simulink model "iPMSM_EKF"  (R2023a)
settings: Solver=FixedStepAuto  StartTime=0.0  StopTime=10  FixedStep=0.0001  RelTol=1e-3  EnableMultiTasking=on
model workspace (MATLAB code in the model file + MAT data in the model file):
  cmdLim = Simulink.Parameter
  cmdLim.Value = 15
  cmdLim.Description = 'Limit for controlling the maximum surface command angle.'
  cmdLim.Min = 0
  cmdLim.Max = 90
  cmdLim.DocUnits = 'deg'
  dispGain = Simulink.Parameter
  dispGain.Value = 0.75
  dispGain.Description = 'Gain applied to the displacement error.'
  dispGain.Min = 0
  dispGain.Max = []
  dispGain.DocUnits = 'deg/sec/deg'
  dispLim = Simulink.Parameter
  dispLim.Value = 30
  dispLim.Description = 'Limit for controlling the maximum commanded angle.'
  dispLim.Min = 0
  dispLim.Max = 180
  dispLim.DocUnits = 'deg'
  intGain = Simulink.Parameter
  intGain.Value = 0.5
  intGain.Description = 'Gain applied to the integral error.'
  intGain.Min = 0
  intGain.Max = []
  intGain.DocUnits = 'deg/sec/deg/sec'
  intLim = Simulink.Parameter
  intLim.Value = 5
  intLim.Description = 'Limit for controlling the maximum commanded angle.'
  intLim.Min = 0
  intLim.Max = 90
  intLim.DocUnits = 'deg'
  rateGain = Simulink.Parameter
  rateGain.Value = 2
  rateGain.Description = 'Gain applied to the rate error.'
  rateGain.Min = 0
  rateGain.Max = []
  rateGain.DocUnits = 'deg/deg/sec'
  rateLim = Simulink.Parameter
  rateLim.Value = 6
  rateLim.Description = 'Limit for controlling the maximum commanded angle.'
  rateLim.Min = 0
  rateLim.Max = 180
  rateLim.DocUnits = 'deg/sec'
  hdgGain = Simulink.Parameter
  hdgGain.Value = 0.015
  VfSvc_EmfEstPiKi_Coef = Simulink.Parameter
  VfSvc_EmfEstPiKi_Coef.Value = 35.163
  VfSvc_EmfEstPiKi_Coef.DataType = 'single'
  VfSvc_EmfEstPiKi_Coef.Complexity = 'real'
  VfSvc_EmfEstPiKi_Coef.Dimensions = [1 1]
  VfSvc_EmfEstPiKp_Coef = Simulink.Parameter
  VfSvc_EmfEstPiKp_Coef.Value = 0.0194
  VfSvc_EmfEstPiKp_Coef.DataType = 'single'
  VfSvc_EmfEstPiKp_Coef.Complexity = 'real'
  VfSvc_EmfEstPiKp_Coef.Dimensions = [1 1]
  VfSvc_eSpeedEstPiKi_Coef = Simulink.Parameter
  VfSvc_eSpeedEstPiKi_Coef.Value = 35.163
  VfSvc_eSpeedEstPiKi_Coef.DataType = 'single'
  VfSvc_eSpeedEstPiKi_Coef.Complexity = 'real'
  VfSvc_eSpeedEstPiKi_Coef.Dimensions = [1 1]
  VfSvc_eSpeedEstPiKp_Coef = Simulink.Parameter
  VfSvc_eSpeedEstPiKp_Coef.Value = 0.0194
  VfSvc_eSpeedEstPiKp_Coef.DataType = 'single'
  VfSvc_eSpeedEstPiKp_Coef.Complexity = 'real'
  VfSvc_eSpeedEstPiKp_Coef.Dimensions = [1 1]
undefined symbols (not defined in the file): DiscIntNeverNeededParam, Flux, ki, kp, Ld, Lq, phi_r, Rs, Ts, We
libraries: slpidlib x2
settings Model: RequirementInfo={} %GIDa_fe9045fd_0412_4b6e_8206_617cc20e6fde  Creator=洲  LastModifiedBy=洲
settings SolverCC: AlgebraicLoopSolver=TrustRegion  AutoInsertRateTranBlk=on
settings DataIOCC: SaveOutput=off  DSMLogging=off  SaveTime=off
settings OptimizationCC: DefaultParameterBehavior=Inlined  UseDivisionForNetSlopeComputation=on  GainParamInheritBuiltInType=on  UseFloatMulNetSlope=on  UseSpecifiedMinMax=on  InlineInvariantSignals=on  EnhancedBackFolding=on  PassReuseOutputArgsAs=Individual arguments  ZeroExternalMemoryAtStartup=off  ZeroInternalMemoryAtStartup=off  NoFixptDivByZeroProtection=on  EfficientFloat2IntCast=on  LifeSpan=1  OptimizeBlockOrder=speed  DifferentSizesBufferReuse=on  OptimizationCustomize=off  EfficientTunableParamExpr=on
settings DebuggingCC: MultiTaskRateTransMsg=warning  AllowSymbolicDim=off  SFUnexpectedBacktrackingDiag=warning  SFNoUnconditionalDefaultTransitionDiag=warning  SFExecutionAtInitializationDiag=none  ArithmeticOperatorsInVariantConditions=warning
settings HardwareCC: ProdLongLongMode=on
settings SFSimCC: MATLABDynamicMemAlloc=off
settings RTWCC: Description=Embedded Coder  SystemTargetFile=ert.tlc  TemplateMakefile=ert_default_tmf  BuildConfiguration=Faster Runs  DataTypeReplacement=CDataTypesFixedWidth
settings CodeAppCC: ForceParamTrailComments=on  IgnoreCustomStorageClasses=off  OperatorAnnotations=on  SimulinkDataObjDesc=on  SFDataObjDesc=on  CustomSymbolStrGlobalVar=rt$N$M  CustomSymbolStrType=$N$M  CustomSymbolStrFcn=$N$M$F  CustomSymbolStrMacro=$N$M  InsertBlockDesc=on  EnableCustomComments=on  ReqsInCode=on
settings ERTTargetCC: TargetLangStandard=C99 (ISO)  UtilityFuncGeneration=Shared location  MultiwordLength=2048  GenerateSampleERTMain=on  IncludeMdlTerminateFcn=off  CombineSignalStateStructs=on  SuppressErrorStatus=on  SupportAbsoluteTime=off  SupportNonFinite=off  SupportComplex=off  InlinedParameterPlacement=NonHierarchical  ERTCustomFileTemplate=example_file_process.tlc  ERTFilePackagingFormat=CompactWithDataFile
settings ConfigComp: CovScope=ReferencedModels  CovSaveName=covdata_rollAP  CovMetricSettings=dcmtrwe  CovHTMLOptions=-sRT=1 -aTS=1 -bRG=1 -bTC=1 -hTR=1 -nFC=0 -scm=1 -bcm=1 -xEv=0  CovSaveCumulativeToWorkspaceVar=on  CovSaveSingleToWorkspaceVar=on  CovCumulativeVarName=covCumulativeData_rollAP  CovReportOnPause=off  CovExternalEMLEnable=off  CovSFcnEnable=off

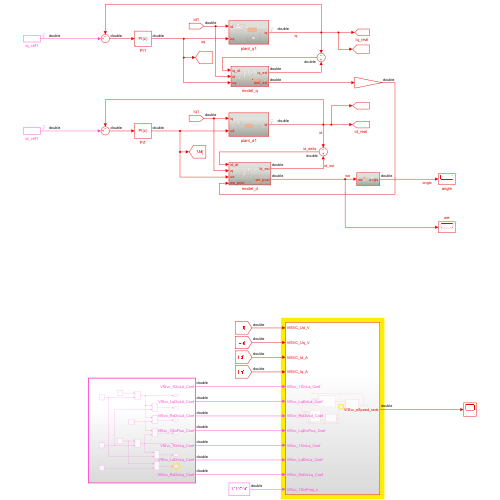
[thumbnail: Simulink's stored preview of the top-level diagram]
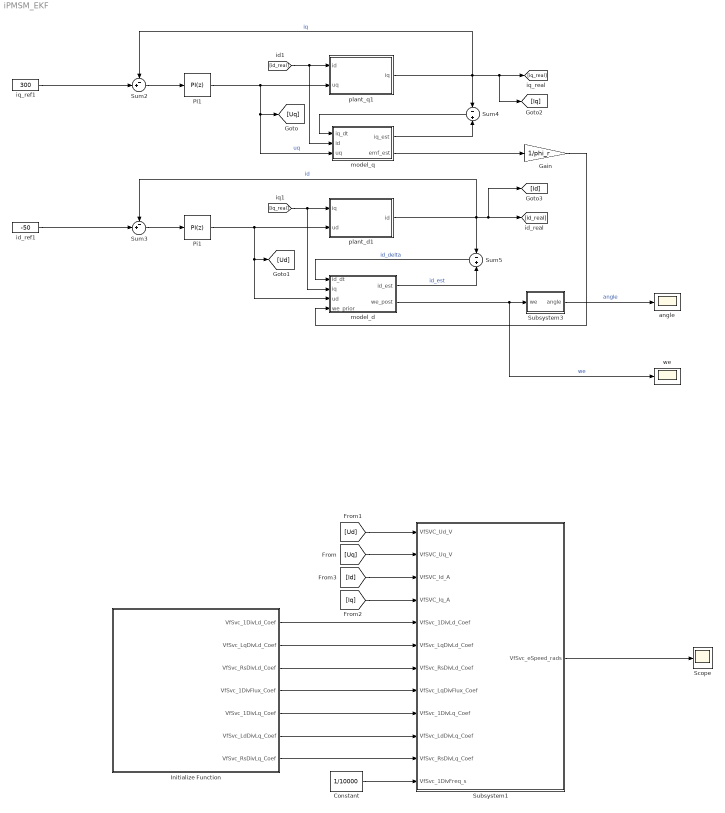
== system iPMSM_EKF ==
  Constant : Constant  Value=1/10000
  Gain : Gain  Gain=1/phi_r
  Initialize Function : Subsystem  TreatAsAtomicUnit=on
  PI1 : slpidlib/PID Controller  Controller=PI  Form=Parallel  TimeDomain=Discrete-time  UseExternalTs=off  SampleTime=-1  IntegratorMethod=Forward Euler  FilterMethod=Forward Euler  ControllerParametersSource=internal  P=1  I=50  UseKiTs=off  D=0  N=100  UseFilter=on  TunerSelectOption=Transfer Function Based (PID Tuner App)  InitialConditionSource=internal  InitialConditionForIntegrator=0  InitialConditionForFilter=0  DifferentiatorICPrevScaledInput=0  ExternalReset=none  TrackingMode=off  Kt=1  LimitOutput=off  SatLimitsSource=internal  UpperSaturationLimit=inf  LowerSaturationLimit=-inf  LinearizeAsGain=on  AntiWindupMode=none  Kb=1  LimitIntegrator=off  UpperIntegratorSaturationLimit=inf  LowerIntegratorSaturationLimit=-inf  POutMin=[]  POutMax=[]  IOutMin=[]  IOutMax=[]  DOutMin=[]  DOutMax=[]  NOutMin=[]  NOutMax=[]  SumOutMin=[]  SumOutMax=[]  SaturationOutMin=[]  SaturationOutMax=[]  PParamMin=[]  PParamMax=[]  IParamMin=[]  IParamMax=[]  DParamMin=[]  DParamMax=[]  NParamMin=[]  NParamMax=[]  KbParamMin=[]  KbParamMax=[]  KtParamMin=[]  KtParamMax=[]  KbOutMin=[]  KbOutMax=[]  KtOutMin=[]  KtOutMax=[]  IntegratorOutMin=[]  IntegratorOutMax=[]  FilterOutMin=[]  FilterOutMax=[]  SumI1OutMin=[]  SumI1OutMax=[]  SumI2OutMin=[]  SumI2OutMax=[]  SumI3OutMin=[]  SumI3OutMax=[]  SumI4OutMin=[]  SumI4OutMax=[]  SumDOutMin=[]  SumDOutMax=[]  DifferentiatorOutMin=[]  DifferentiatorOutMax=[]  FilterDiffOutCoefMin=[]  FilterDiffOutCoefMax=[]  ReciprocalOutMin=[]  ReciprocalOutMax=[]  SumDenOutMin=[]  SumDenOutMax=[]  SumNumOutMin=[]  SumNumOutMax=[]  DivideOutMin=[]  DivideOutMax=[]  UdiffTsProdOutMin=[]  UdiffTsProdOutMax=[]  NTsProdOutMin=[]  NTsProdOutMax=[]  UintegralTsProdOutMin=[]  UintegralTsProdOutMax=[]  UngainTsProdOutMin=[]  UngainTsProdOutMax=[]  ClampingZeroOutDataTypeStr=Inherit: Inherit via back propagation  ClampingZeroOutMin=[]  ClampingZeroOutMax=[]  FilterDenConstantOutDataTypeStr=Inherit: Inherit via back propagation  FilterDenConstantOutMin=[]  FilterDenConstantOutMax=[]  PCopyOutDataTypeStr=Inherit: Inherit via back propagation  PCopyOutMin=[]  PCopyOutMax=[]  NCopyOutDataTypeStr=Inherit: Inherit via back propagation  NCopyOutMin=[]  NCopyOutMax=[]  IntegratorContinuousStateAttributes=''  IntegratorStateMustResolveToSignalObject=off  IntegratorRTWStateStorageClass=Auto  FilterContinuousStateAttributes=''  FilterStateMustResolveToSignalObject=off  FilterRTWStateStorageClass=Auto  ParallelPVariant=InternalParameters  IdealPVariant=Disabled  IVariant=InternalParameters  DVariant=Disabled  IntegratorVariant=Discrete  SatVariant=Disabled  AWVariant=Passthrough  PCopyVariant=Disabled  TRVariant=Disabled  FdbkBlocksVariant=Forward  IdealPFdbkVariant=Disabled  SatFdbkVariant=Disabled  DerivativeFilterVariant=Disabled  NVariant=Disabled  NCopyVariant=Disabled_SignalSpec  FilterICVariant=Disabled  IntegratorICVariant=InternalICs  ExternalResetVariant=Disabled  TRSumVariant=Passthrough  SumFdbkVariant=Disabled  SumVariant=Sum_PI  TsampFilterVariant=InternalTs  TsampNgainVariant=Passthrough  TsampIntegralVariant=Disabled_SignalSpec  ExternalSaturationOutDataTypeStr=Inherit: Same as second input
  Pi1 : slpidlib/PID Controller  Controller=PI  Form=Parallel  TimeDomain=Discrete-time  UseExternalTs=off  SampleTime=-1  IntegratorMethod=Forward Euler  FilterMethod=Forward Euler  ControllerParametersSource=internal  P=1  I=50  UseKiTs=off  D=0  N=100  UseFilter=on  TunerSelectOption=Transfer Function Based (PID Tuner App)  InitialConditionSource=internal  InitialConditionForIntegrator=0  InitialConditionForFilter=0  DifferentiatorICPrevScaledInput=0  ExternalReset=none  TrackingMode=off  Kt=1  LimitOutput=off  SatLimitsSource=internal  UpperSaturationLimit=inf  LowerSaturationLimit=-inf  LinearizeAsGain=on  AntiWindupMode=none  Kb=1  LimitIntegrator=off  UpperIntegratorSaturationLimit=inf  LowerIntegratorSaturationLimit=-inf  POutMin=[]  POutMax=[]  IOutMin=[]  IOutMax=[]  DOutMin=[]  DOutMax=[]  NOutMin=[]  NOutMax=[]  SumOutMin=[]  SumOutMax=[]  SaturationOutMin=[]  SaturationOutMax=[]  PParamMin=[]  PParamMax=[]  IParamMin=[]  IParamMax=[]  DParamMin=[]  DParamMax=[]  NParamMin=[]  NParamMax=[]  KbParamMin=[]  KbParamMax=[]  KtParamMin=[]  KtParamMax=[]  KbOutMin=[]  KbOutMax=[]  KtOutMin=[]  KtOutMax=[]  IntegratorOutMin=[]  IntegratorOutMax=[]  FilterOutMin=[]  FilterOutMax=[]  SumI1OutMin=[]  SumI1OutMax=[]  SumI2OutMin=[]  SumI2OutMax=[]  SumI3OutMin=[]  SumI3OutMax=[]  SumI4OutMin=[]  SumI4OutMax=[]  SumDOutMin=[]  SumDOutMax=[]  DifferentiatorOutMin=[]  DifferentiatorOutMax=[]  FilterDiffOutCoefMin=[]  FilterDiffOutCoefMax=[]  ReciprocalOutMin=[]  ReciprocalOutMax=[]  SumDenOutMin=[]  SumDenOutMax=[]  SumNumOutMin=[]  SumNumOutMax=[]  DivideOutMin=[]  DivideOutMax=[]  UdiffTsProdOutMin=[]  UdiffTsProdOutMax=[]  NTsProdOutMin=[]  NTsProdOutMax=[]  UintegralTsProdOutMin=[]  UintegralTsProdOutMax=[]  UngainTsProdOutMin=[]  UngainTsProdOutMax=[]  ClampingZeroOutDataTypeStr=Inherit: Inherit via back propagation  ClampingZeroOutMin=[]  ClampingZeroOutMax=[]  FilterDenConstantOutDataTypeStr=Inherit: Inherit via back propagation  FilterDenConstantOutMin=[]  FilterDenConstantOutMax=[]  PCopyOutDataTypeStr=Inherit: Inherit via back propagation  PCopyOutMin=[]  PCopyOutMax=[]  NCopyOutDataTypeStr=Inherit: Inherit via back propagation  NCopyOutMin=[]  NCopyOutMax=[]  IntegratorContinuousStateAttributes=''  IntegratorStateMustResolveToSignalObject=off  IntegratorRTWStateStorageClass=Auto  FilterContinuousStateAttributes=''  FilterStateMustResolveToSignalObject=off  FilterRTWStateStorageClass=Auto  ParallelPVariant=InternalParameters  IdealPVariant=Disabled  IVariant=InternalParameters  DVariant=Disabled  IntegratorVariant=Discrete  SatVariant=Disabled  AWVariant=Passthrough  PCopyVariant=Disabled  TRVariant=Disabled  FdbkBlocksVariant=Forward  IdealPFdbkVariant=Disabled  SatFdbkVariant=Disabled  DerivativeFilterVariant=Disabled  NVariant=Disabled  NCopyVariant=Disabled_SignalSpec  FilterICVariant=Disabled  IntegratorICVariant=InternalICs  ExternalResetVariant=Disabled  TRSumVariant=Passthrough  SumFdbkVariant=Disabled  SumVariant=Sum_PI  TsampFilterVariant=InternalTs  TsampNgainVariant=Passthrough  TsampIntegralVariant=Disabled_SignalSpec  ExternalSaturationOutDataTypeStr=Inherit: Same as second input
  Scope : Scope
  Subsystem1 : Subsystem
  Subsystem3 : Subsystem
  Sum2 : Sum  Inputs=-+|
  Sum3 : Sum  Inputs=-+|
  Sum4 : Sum  Inputs=-+
  Sum5 : Sum  Inputs=-+
  angle : Scope
  id_ref1 : Constant  Value=-50
  iq_ref1 : Constant  Value=300
  model_d : Subsystem
  model_q : Subsystem
  plant_d1 : Subsystem
  plant_q1 : Subsystem
  we : Scope
  wires:
  Initialize Function/1(VfSvc_1DivLd_Coef) -> Subsystem1/5(VfSvc_1DivLd_Coef)
  Initialize Function/2(VfSvc_LqDivLd_Coef) -> Subsystem1/6(VfSvc_LqDivLd_Coef)
  Initialize Function/3(VfSvc_RsDivLd_Coef) -> Subsystem1/7(VfSvc_RsDivLd_Coef)
  Initialize Function/5(VfSvc_1DivLq_Coef) -> Subsystem1/9(VfSvc_1DivLq_Coef)
  Initialize Function/6(VfSvc_LdDivLq_Coef) -> Subsystem1/10(VfSvc_LdDivLq_Coef)
  Initialize Function/7(VfSvc_RsDivLq_Coef) -> Subsystem1/11(VfSvc_RsDivLq_Coef)
  Initialize Function/4(VfSvc_1DivFlux_Coef) -> Subsystem1/8(VfSvc_LqDivFlux_Coef)
  Constant/1 -> Subsystem1/12(VfSvc_1DivFreq_s)
  Subsystem1/1(VfSvc_eSpeed_rads) -> Scope/1
  model_d/1(id_est) -> Sum5/2  "id_est"
  plant_q1/1(iq) -> Sum2/1, [Iq], [iq_real], Sum4/1  "iq"
  plant_d1/1(id) -> Sum3/1, Sum5/1, [Id], [id_real]  "id"
  Subsystem3/1(angle) -> angle/1  "angle"
  Sum2/1 -> PI1/1
  model_d/2(we_post) -> we/1, Subsystem3/1(we)  "we"
  iq_ref1/1 -> Sum2/2
  Gain/1 -> model_d/4(we_prior)
  Pi1/1 -> [Ud], model_d/3(ud), plant_d1/2(ud)
  Sum5/1 -> model_d/1(id_dt)  "id_delta"
  id_ref1/1 -> Sum3/2
  model_q/2(emf_est) -> Gain/1
  Sum4/1 -> model_q/1(iq_dt)
  [iq_real] -> plant_d1/1(iq), model_d/2(iq)
  [id_real] -> model_q/2(id), plant_q1/1(id)
  PI1/1 -> plant_q1/2(uq), model_q/3(uq), [Uq]  "uq"
  Sum3/1 -> Pi1/1
  model_q/1(iq_est) -> Sum4/2
  [Uq] -> Subsystem1/2(VfSVC_Uq_V)
  [Ud] -> Subsystem1/1(VfSVC_Ud_V)
  [Id] -> Subsystem1/3(VfSVC_Id_A)
  [Iq] -> Subsystem1/4(VfSVC_Iq_A)

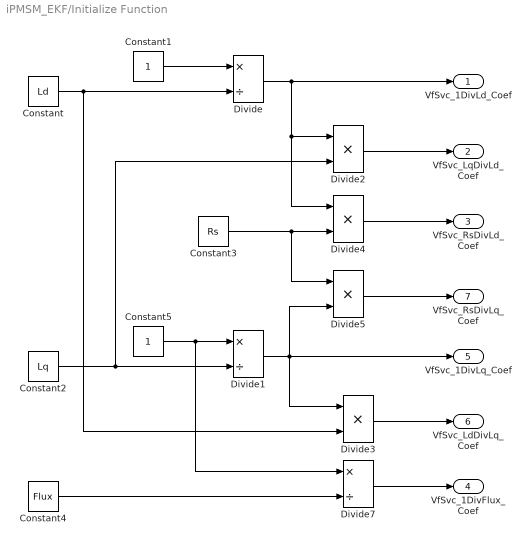
== system iPMSM_EKF/Initialize Function ==
  Constant : Constant  Value=Ld
  Constant1 : Constant
  Constant2 : Constant  Value=Lq
  Constant3 : Constant  Value=Rs
  Constant4 : Constant  Value=Flux
  Constant5 : Constant
  Divide : Product  Inputs=*/
  Divide1 : Product  Inputs=*/
  Divide{2..5} (4 alike) : Product  Inputs=**
  Divide7 : Product  Inputs=*/
  VfSvc_1DivLd_Coef : Outport
  VfSvc_LqDivLd_Coef : Outport  Port=2
  VfSvc_RsDivLd_Coef : Outport  Port=3
  VfSvc_1DivFlux_Coef : Outport  Port=4
  VfSvc_1DivLq_Coef : Outport  Port=5
  VfSvc_LdDivLq_Coef : Outport  Port=6
  VfSvc_RsDivLq_Coef : Outport  Port=7
  wires:
  Constant1/1 -> Divide/1
  Divide/1 -> Divide4/1, Divide2/1, VfSvc_1DivLd_Coef/1
  Constant5/1 -> Divide7/1, Divide1/1
  Divide2/1 -> VfSvc_LqDivLd_Coef/1
  Divide1/1 -> Divide5/2, Divide3/1, VfSvc_1DivLq_Coef/1
  Divide3/1 -> VfSvc_LdDivLq_Coef/1
  Constant/1 -> Divide3/2, Divide/2
  Constant3/1 -> Divide5/1, Divide4/2
  Divide4/1 -> VfSvc_RsDivLd_Coef/1
  Divide5/1 -> VfSvc_RsDivLq_Coef/1
  Constant4/1 -> Divide7/2
  Constant2/1 -> Divide1/2, Divide2/2
  Divide7/1 -> VfSvc_1DivFlux_Coef/1

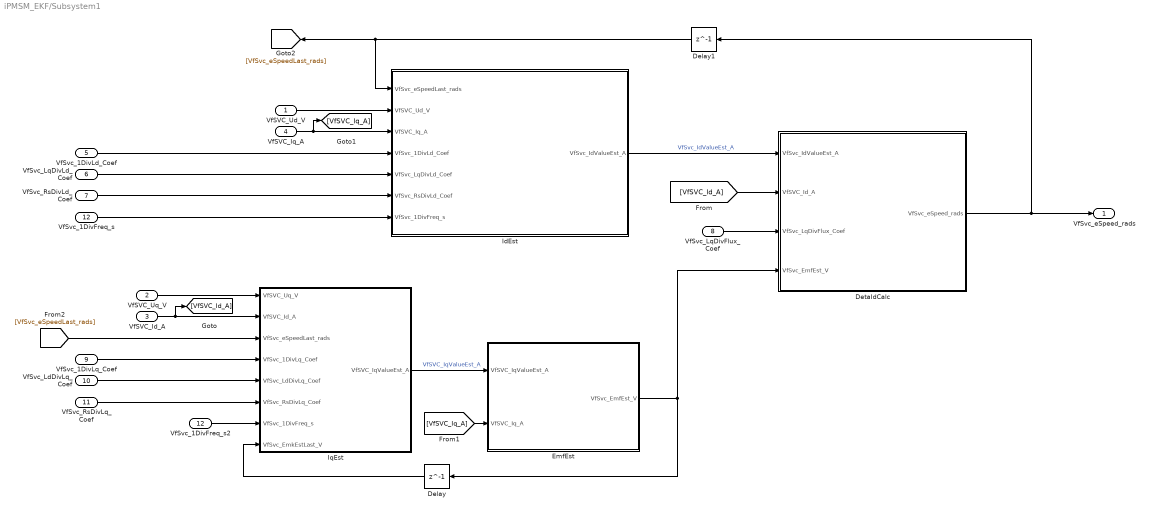
== system iPMSM_EKF/Subsystem1 ==
  VfSVC_Ud_V : Inport
  VfSVC_Uq_V : Inport  Port=2
  VfSVC_Id_A : Inport  Port=3
  VfSVC_Iq_A : Inport  Port=4
  VfSvc_1DivLd_Coef : Inport  Port=5
  VfSvc_LqDivLd_Coef : Inport  Port=6
  VfSvc_RsDivLd_Coef : Inport  Port=7
  VfSvc_LqDivFlux_Coef : Inport  Port=8
  VfSvc_1DivLq_Coef : Inport  Port=9
  VfSvc_LdDivLq_Coef : Inport  Port=10
  VfSvc_RsDivLq_Coef : Inport  Port=11
  VfSvc_1DivFreq_s : Inport  Port=12
  Delay : Delay  DelayLength=1
  Delay1 : Delay  DelayLength=1
  DetaIdCalc : Subsystem
  EmfEst : Subsystem
  IdEst : Subsystem
  IqEst : Subsystem
  VfSvc_1DivFreq_s2 : InportShadow  Port=12
  VfSvc_eSpeed_rads : Outport
  wires:
  VfSVC_Iq_A/1 -> [VfSVC_Iq_A], IdEst/3(VfSVC_Iq_A)
  DetaIdCalc/1(VfSvc_eSpeed_rads) -> Delay1/1, VfSvc_eSpeed_rads/1
  VfSvc_1DivLq_Coef/1 -> IqEst/4(VfSvc_1DivLq_Coef)
  [VfSVC_Iq_A] -> EmfEst/2(VfSVC_Iq_A)
  VfSVC_Uq_V/1 -> IqEst/1(VfSVC_Uq_V)
  Delay1/1 -> [VfSvc_eSpeedLast_rads], IdEst/1(VfSvc_eSpeedLast_rads)
  VfSVC_Id_A/1 -> IqEst/2(VfSVC_Id_A), [VfSVC_Id_A]
  EmfEst/1(VfSvc_EmfEst_V) -> DetaIdCalc/4(VfSvc_EmfEst_V), Delay/1
  Delay/1 -> IqEst/8(VfSvc_EmkEstLast_V)
  IdEst/1(VfSvc_IdValueEst_A) -> DetaIdCalc/1(VfSvc_IdValueEst_A)  "VfSvc_IdValueEst_A"
  VfSvc_LqDivFlux_Coef/1 -> DetaIdCalc/3(VfSvc_LqDivFlux_Coef)
  VfSVC_Ud_V/1 -> IdEst/2(VfSVC_Ud_V)
  [VfSVC_Id_A] -> DetaIdCalc/2(VfSVC_Id_A)
  VfSvc_RsDivLq_Coef/1 -> IqEst/6(VfSvc_RsDivLq_Coef)
  IqEst/1(VfSVC_IqValueEst_A) -> EmfEst/1(VfSVC_IqValueEst_A)  "VfSVC_IqValueEst_A"
  VfSvc_1DivFreq_s/1 -> IdEst/7(VfSvc_1DivFreq_s)
  VfSvc_LqDivLd_Coef/1 -> IdEst/5(VfSvc_LqDivLd_Coef)
  VfSvc_1DivLd_Coef/1 -> IdEst/4(VfSvc_1DivLd_Coef)
  VfSvc_LdDivLq_Coef/1 -> IqEst/5(VfSvc_LdDivLq_Coef)
  VfSvc_RsDivLd_Coef/1 -> IdEst/6(VfSvc_RsDivLd_Coef)
  VfSvc_1DivFreq_s2/1 -> IqEst/7(VfSvc_1DivFreq_s)
  [VfSvc_eSpeedLast_rads] -> IqEst/3(VfSvc_eSpeedLast_rads)

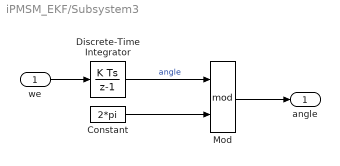
== system iPMSM_EKF/Subsystem3 ==
  we : Inport
  Constant : Constant  Value=2*pi
  Discrete-Time Integrator : DiscreteIntegrator  SampleTime=-1  ICPrevOutput=DiscIntNeverNeededParam  ICPrevScaledInput=DiscIntNeverNeededParam
  Mod : Math  Operator=mod  SignedPower=on
  angle : Outport  VectorParamsAs1DForOutWhenUnconnected=off
  wires:
  Constant/1 -> Mod/2
  we/1 -> Discrete-Time Integrator/1
  Mod/1 -> angle/1
  Discrete-Time Integrator/1 -> Mod/1  "angle"

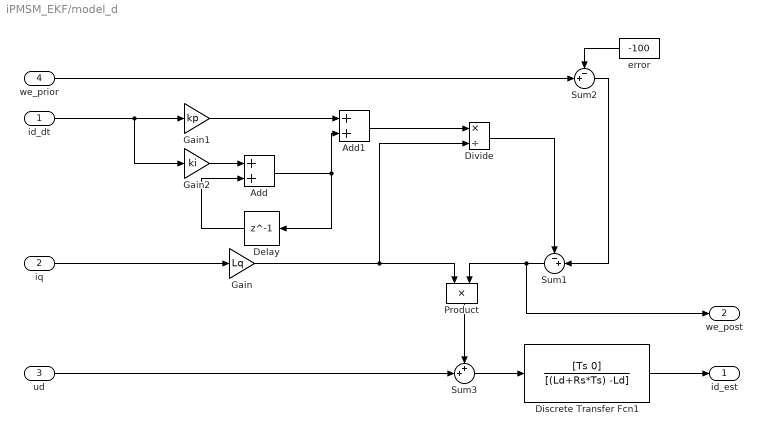
== system iPMSM_EKF/model_d ==
  id_dt : Inport
  iq : Inport  Port=2
  ud : Inport  Port=3
  we_prior : Inport  Port=4
  Add : Sum
  Add1 : Sum
  Delay : Delay  DelayLength=1
  Discrete Transfer Fcn1 : DiscreteTransferFcn  Numerator=[Ts 0]  Denominator=[(Ld+Rs*Ts) -Ld]
  Divide : Product  Inputs=*/
  Gain : Gain  Gain=Lq
  Gain1 : Gain  Gain=kp
  Gain2 : Gain  Gain=ki
  Product : Product
  Sum1 : Sum  Inputs=-+|
  Sum2 : Sum  Inputs=-+|
  Sum3 : Sum  Inputs=++|
  error : Constant  Value=-100
  id_est : Outport  VectorParamsAs1DForOutWhenUnconnected=off
  we_post : Outport  Port=2  VectorParamsAs1DForOutWhenUnconnected=off
  wires:
  iq/1 -> Gain/1
  ud/1 -> Sum3/2
  Sum3/1 -> Discrete Transfer Fcn1/1
  Gain/1 -> Product/1, Divide/2
  Product/1 -> Sum3/1
  Sum1/1 -> Product/2, we_post/1
  we_prior/1 -> Sum2/2
  error/1 -> Sum2/1
  Sum2/1 -> Sum1/2
  Discrete Transfer Fcn1/1 -> id_est/1
  id_dt/1 -> Gain2/1, Gain1/1
  Divide/1 -> Sum1/1
  Gain1/1 -> Add1/1
  Gain2/1 -> Add/1
  Add/1 -> Delay/1, Add1/2
  Delay/1 -> Add/2
  Add1/1 -> Divide/1

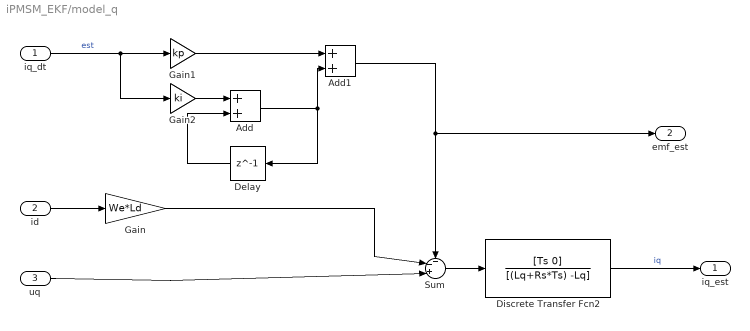
== system iPMSM_EKF/model_q ==
  iq_dt : Inport
  id : Inport  Port=2
  uq : Inport  Port=3
  Add : Sum
  Add1 : Sum
  Delay : Delay  DelayLength=1
  Discrete Transfer Fcn2 : DiscreteTransferFcn  Numerator=[Ts 0]  Denominator=[(Lq+Rs*Ts) -Lq]
  Gain : Gain  Gain=We*Ld
  Gain1 : Gain  Gain=kp
  Gain2 : Gain  Gain=ki
  Sum : Sum  Inputs=--+|
  iq_est : Outport  VectorParamsAs1DForOutWhenUnconnected=off
  emf_est : Outport  Port=2  VectorParamsAs1DForOutWhenUnconnected=off
  wires:
  iq_dt/1 -> Gain1/1, Gain2/1  "est"
  Gain/1 -> Sum/2
  uq/1 -> Sum/3
  Sum/1 -> Discrete Transfer Fcn2/1
  Add1/1 -> emf_est/1, Sum/1
  Discrete Transfer Fcn2/1 -> iq_est/1  "iq"
  id/1 -> Gain/1
  Delay/1 -> Add/2
  Gain1/1 -> Add1/1
  Gain2/1 -> Add/1
  Add/1 -> Delay/1, Add1/2

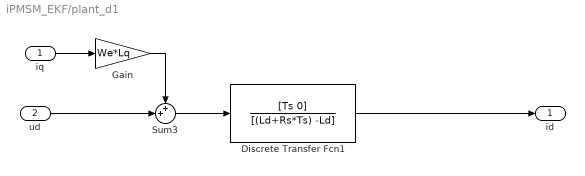
== system iPMSM_EKF/plant_d1 ==
  iq : Inport
  ud : Inport  Port=2
  Discrete Transfer Fcn1 : DiscreteTransferFcn  Numerator=[Ts 0]  Denominator=[(Ld+Rs*Ts) -Ld]
  Gain : Gain  Gain=We*Lq
  Sum3 : Sum  Inputs=++|
  id : Outport  VectorParamsAs1DForOutWhenUnconnected=off
  wires:
  iq/1 -> Gain/1
  ud/1 -> Sum3/2
  Sum3/1 -> Discrete Transfer Fcn1/1
  Gain/1 -> Sum3/1
  Discrete Transfer Fcn1/1 -> id/1

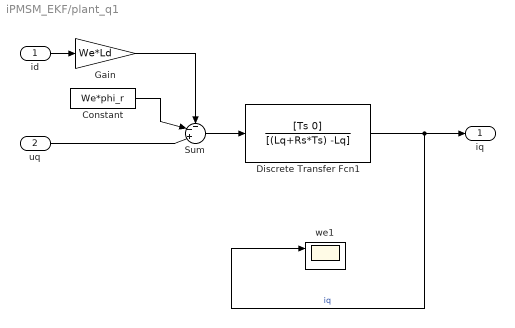
== system iPMSM_EKF/plant_q1 ==
  id : Inport
  uq : Inport  Port=2
  Constant : Constant  Value=We*phi_r
  Discrete Transfer Fcn1 : DiscreteTransferFcn  Numerator=[Ts 0]  Denominator=[(Lq+Rs*Ts) -Lq]
  Gain : Gain  Gain=We*Ld
  Sum : Sum  Inputs=--+|
  we1 : Scope  NumInputPorts=2
  iq : Outport  VectorParamsAs1DForOutWhenUnconnected=off
  wires:
  id/1 -> Gain/1
  Discrete Transfer Fcn1/1 -> we1/1, iq/1  "iq"
  Sum/1 -> Discrete Transfer Fcn1/1
  uq/1 -> Sum/3
  Gain/1 -> Sum/1
  Constant/1 -> Sum/2

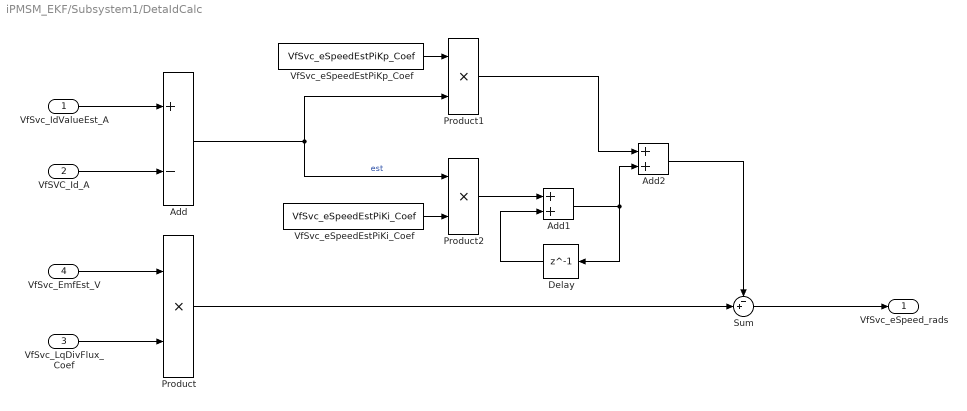
== system iPMSM_EKF/Subsystem1/DetaIdCalc ==
  VfSvc_IdValueEst_A : Inport
  VfSVC_Id_A : Inport  Port=2
  VfSvc_LqDivFlux_Coef : Inport  Port=3
  VfSvc_EmfEst_V : Inport  Port=4
  Add : Sum  Inputs=+-
  Add1 : Sum
  Add2 : Sum
  Delay : Delay  DelayLength=1
  Product : Product
  Product1 : Product
  Product2 : Product
  Sum : Sum  Inputs=-+|
  VfSvc_eSpeedEstPiKi_Coef : Constant  Value=VfSvc_eSpeedEstPiKi_Coef
  VfSvc_eSpeedEstPiKp_Coef : Constant  Value=VfSvc_eSpeedEstPiKp_Coef
  VfSvc_eSpeed_rads : Outport
  wires:
  VfSvc_IdValueEst_A/1 -> Add/1
  VfSVC_Id_A/1 -> Add/2
  Product1/1 -> Add2/1
  Delay/1 -> Add1/2
  Add/1 -> Product1/2, Product2/1  "est"
  Add1/1 -> Delay/1, Add2/2
  Product2/1 -> Add1/1
  VfSvc_EmfEst_V/1 -> Product/1
  VfSvc_LqDivFlux_Coef/1 -> Product/2
  Product/1 -> Sum/2
  Add2/1 -> Sum/1
  Sum/1 -> VfSvc_eSpeed_rads/1
  VfSvc_eSpeedEstPiKp_Coef/1 -> Product1/1
  VfSvc_eSpeedEstPiKi_Coef/1 -> Product2/2

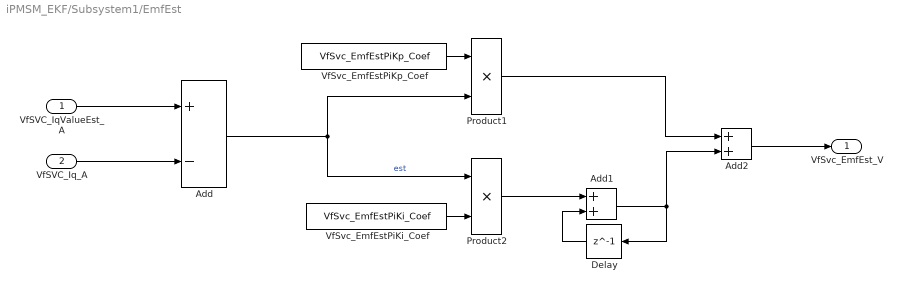
== system iPMSM_EKF/Subsystem1/EmfEst ==
  VfSVC_IqValueEst_A : Inport
  VfSVC_Iq_A : Inport  Port=2
  Add : Sum  Inputs=+-
  Add1 : Sum
  Add2 : Sum
  Delay : Delay  DelayLength=1
  Product1 : Product
  Product2 : Product
  VfSvc_EmfEstPiKi_Coef : Constant  Value=VfSvc_EmfEstPiKi_Coef
  VfSvc_EmfEstPiKp_Coef : Constant  Value=VfSvc_EmfEstPiKp_Coef
  VfSvc_EmfEst_V : Outport
  wires:
  VfSVC_IqValueEst_A/1 -> Add/1
  VfSVC_Iq_A/1 -> Add/2
  Add2/1 -> VfSvc_EmfEst_V/1
  VfSvc_EmfEstPiKp_Coef/1 -> Product1/1
  Add/1 -> Product2/1, Product1/2  "est"
  VfSvc_EmfEstPiKi_Coef/1 -> Product2/2
  Product2/1 -> Add1/1
  Product1/1 -> Add2/1
  Add1/1 -> Delay/1, Add2/2
  Delay/1 -> Add1/2

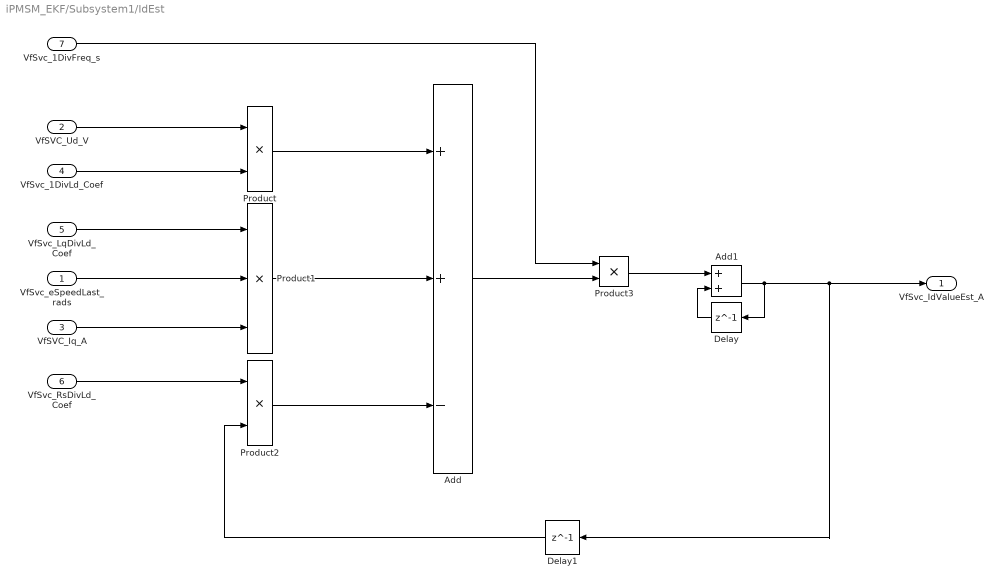
== system iPMSM_EKF/Subsystem1/IdEst ==
  VfSvc_eSpeedLast_rads : Inport
  VfSVC_Ud_V : Inport  Port=2
  VfSVC_Iq_A : Inport  Port=3
  VfSvc_1DivLd_Coef : Inport  Port=4
  VfSvc_LqDivLd_Coef : Inport  Port=5
  VfSvc_RsDivLd_Coef : Inport  Port=6
  VfSvc_1DivFreq_s : Inport  Port=7
  Add : Sum  Inputs=++-
  Add1 : Sum
  Delay : Delay  DelayLength=1
  Delay1 : Delay  DelayLength=1
  Product : Product
  Product1 : Product  Inputs=3
  Product2 : Product
  Product3 : Product
  VfSvc_IdValueEst_A : Outport
  wires:
  VfSVC_Ud_V/1 -> Product/1
  VfSvc_1DivLd_Coef/1 -> Product/2
  VfSvc_LqDivLd_Coef/1 -> Product1/1
  VfSvc_eSpeedLast_rads/1 -> Product1/2
  VfSVC_Iq_A/1 -> Product1/3
  VfSvc_RsDivLd_Coef/1 -> Product2/1
  Product/1 -> Add/1
  Product1/1 -> Add/2
  Product2/1 -> Add/3
  Add/1 -> Product3/2
  VfSvc_1DivFreq_s/1 -> Product3/1
  Product3/1 -> Add1/1
  Add1/1 -> Delay1/1, VfSvc_IdValueEst_A/1, Delay/1
  Delay/1 -> Add1/2
  Delay1/1 -> Product2/2

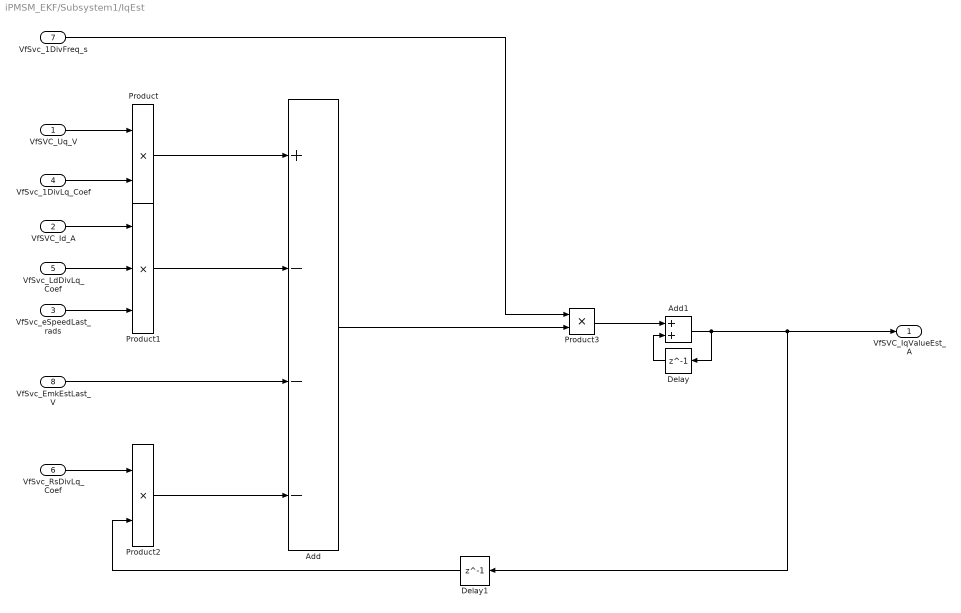
== system iPMSM_EKF/Subsystem1/IqEst ==
  VfSVC_Uq_V : Inport
  VfSVC_Id_A : Inport  Port=2
  VfSvc_eSpeedLast_rads : Inport  Port=3
  VfSvc_1DivLq_Coef : Inport  Port=4
  VfSvc_LdDivLq_Coef : Inport  Port=5
  VfSvc_RsDivLq_Coef : Inport  Port=6
  VfSvc_1DivFreq_s : Inport  Port=7
  VfSvc_EmkEstLast_V : Inport  Port=8
  Add : Sum  Inputs=+---
  Add1 : Sum
  Delay : Delay  DelayLength=1
  Delay1 : Delay  DelayLength=1
  Product : Product
  Product1 : Product  Inputs=3
  Product2 : Product
  Product3 : Product
  VfSVC_IqValueEst_A : Outport
  wires:
  VfSVC_Uq_V/1 -> Product/1
  VfSvc_1DivLq_Coef/1 -> Product/2
  VfSvc_LdDivLq_Coef/1 -> Product1/2
  VfSvc_eSpeedLast_rads/1 -> Product1/3
  VfSVC_Id_A/1 -> Product1/1
  VfSvc_RsDivLq_Coef/1 -> Product2/1
  Product/1 -> Add/1
  Product1/1 -> Add/2
  VfSvc_EmkEstLast_V/1 -> Add/3
  Product2/1 -> Add/4
  Delay/1 -> Add1/2
  Add1/1 -> Delay1/1, VfSVC_IqValueEst_A/1, Delay/1
  VfSvc_1DivFreq_s/1 -> Product3/1
  Product3/1 -> Add1/1
  Add/1 -> Product3/2
  Delay1/1 -> Product2/2
